simulink library "component_lib"  (R2023a)
settings: Solver=VariableStepAuto  StartTime=0.0  StopTime=10.0  RelTol=1e-3
undefined symbols (not defined in the file or in its folder): ECCV_r, par, R1234yf_ph, V_nom
libraries: base_lib x258, $bdroot x212, simulink x2, slpidlib x1
(part 5 of 7)

== system component_lib/Thermal Systems/RF0003_compressor ==
  V_bus [V] : Inport
  p2 [Pa] : Inport  Port=2
  N [rpm] : Inport  Port=3
  "RF: (h1, p1, ~)" : Inport  Port=4
  Constant : Constant  Value=W0
  Constant1 : Constant  Value=400e3
  Demux : Demux  Outputs=3
  Density Look-up : Lookup_n-D  BreakpointsForDimension1=R1234yf_ph.p  BreakpointsForDimension2=R1234yf_ph.h  Table=R1234yf_ph.D  InternalRulePriority=Speed  RndMeth=Simplest
      settings: InputPortMap=u0,u1
  Divide : Product  Inputs=*/
  Divide1 : Product  Inputs=*/
  F0021_cp.m : base_lib/F0021_R1234yf/F0021_cp.m  SystemSampleTime=-1  VariantActivationTime=update diagram  Latency=0  AutoFrameSizeCalculation=off
      settings: LibrarySourceBlock=|
      | simulink/User-Defined
      | Functions/MATLAB Function
  F0021_cv.m : base_lib/F0021_R1234yf/F0021_cv.m  SystemSampleTime=-1  VariantActivationTime=update diagram  Latency=0  AutoFrameSizeCalculation=off
      settings: LibrarySourceBlock=|
      | simulink/User-Defined
      | Functions/MATLAB Function
  F0022_compressor.m : base_lib/F0022_heatPump/F0022_compressor.m  SystemSampleTime=-1  VariantActivationTime=update diagram  Latency=0  AutoFrameSizeCalculation=off
      settings: LibrarySourceBlock=|
      | simulink/User-Defined
      | Functions/MATLAB Function
  Gain : Gain  Gain=1/60
  Gain1 : Gain  Gain=par.M
  Gain2 : Gain  Gain=1/par.M
  Gain3 : Gain  Gain=1/t_c
  Gain4 : Gain  Gain=1/t_c
  Integrator : Integrator  InitialConditionSource=external  LimitOutput=on  LowerSaturationLimit=0
  Integrator1 : Integrator  InitialConditionSource=external  LimitOutput=on  LowerSaturationLimit=0
  Mux : Mux  Inputs=3
  Negative flow barred : Saturate  UpperLimit=inf  LowerLimit=0
  Power limit : Saturate  UpperLimit=1e4  LowerLimit=0
  Saturation : Saturate  UpperLimit=par.Tc-1  LowerLimit=0
  Sum : Sum  Inputs=|+-
  Sum1 : Sum  Inputs=|+-
  Temperature Look-up : Lookup_n-D  BreakpointsForDimension1=R1234yf_ph.p  BreakpointsForDimension2=R1234yf_ph.h  Table=R1234yf_ph.T  InternalRulePriority=Speed  RndMeth=Simplest
      settings: InputPortMap=u0,u1
  Terminator : Terminator
  I [A] : Outport
  "RF: (h2, p2, W2)" : Outport  Port=2
  wires:
  Gain1/1 -> F0022_compressor.m/3, Density Look-up/2, Temperature Look-up/2
  [p_1] -> Temperature Look-up/1, Density Look-up/1, F0022_compressor.m/1
  N [rpm]/1 -> Gain/1
  F0022_compressor.m/1 -> Negative flow barred/1
  F0022_compressor.m/2 -> Power limit/1
  Density Look-up/1 -> F0022_compressor.m/2, F0021_cv.m/2, F0021_cp.m/2
  F0021_cp.m/1 -> Divide/1
  F0021_cv.m/1 -> Divide/2
  Divide/1 -> F0022_compressor.m/6
  Temperature Look-up/1 -> Saturation/1
  F0022_compressor.m/3 -> Gain2/1
  p2 [Pa]/1 -> [p_2], F0022_compressor.m/4
  Saturation/1 -> F0021_cv.m/1, F0021_cp.m/1
  Negative flow barred/1 -> Sum/1
  Gain/1 -> F0022_compressor.m/5
  Integrator/1 -> Sum/2, [W]
  [h_1] -> Gain1/1
  "RF: (h1, p1, ~)"/1 -> Demux/1
  Demux/1 -> [h_1]
  Demux/2 -> [p_1]
  Mux/1 -> "RF: (h2, p2, W2)"/1
  [h_2] -> Mux/1
  [p_2] -> Mux/2
  [W] -> Mux/3
  Demux/3 -> Terminator/1
  Sum/1 -> Gain3/1
  Gain3/1 -> Integrator/1
  Constant/1 -> Integrator/2
  Gain2/1 -> Sum1/1
  Sum1/1 -> Gain4/1
  Integrator1/1 -> Sum1/2, [h_2]
  Gain4/1 -> Integrator1/1
  Constant1/1 -> Integrator1/2
  V_bus [V]/1 -> Divide1/2
  Power limit/1 -> Divide1/1
  Divide1/1 -> I [A]/1

== system component_lib/Thermal Systems/RF0004_smoothTube ==
  "RF: (h1, p1, W1)" : Inport
  Abs : Abs  SaturateOnIntegerOverflow=off
  Demux : Demux  Outputs=3
  F0021_dliqsat.m : base_lib/F0021_R1234yf/F0021_dliqsat.m  SystemSampleTime=-1  VariantActivationTime=update diagram  Latency=0  AutoFrameSizeCalculation=off
      settings: LibrarySourceBlock=|
      | simulink/User-Defined
      | Functions/MATLAB Function
  F0021_dvapsat.m : base_lib/F0021_R1234yf/F0021_dvapsat.m  SystemSampleTime=-1  VariantActivationTime=update diagram  Latency=0  AutoFrameSizeCalculation=off
      settings: LibrarySourceBlock=|
      | simulink/User-Defined
      | Functions/MATLAB Function
  F0022_smoothTubePressureDrop.m : base_lib/F0022_heatPump/F0022_smoothTubePressureDrop.m  SystemSampleTime=-1  VariantActivationTime=update diagram  Latency=0  AutoFrameSizeCalculation=off
      settings: LibrarySourceBlock=|
      | simulink/User-Defined
      | Functions/MATLAB Function
  Gain{2,4..5,7} (4 alike) : Gain  Gain=par.M
  Mux : Mux  Inputs=3
  R1234yf_mu.m : base_lib/F0021_R1234yf/R1234yf_mu.m  SystemSampleTime=-1  VariantActivationTime=update diagram  Latency=0  AutoFrameSizeCalculation=off
      settings: LibrarySourceBlock=|
      | simulink/User-Defined
      | Functions/MATLAB Function
  R1234yf_mu.m1 : base_lib/F0021_R1234yf/R1234yf_mu.m  SystemSampleTime=-1  VariantActivationTime=update diagram  Latency=0  AutoFrameSizeCalculation=off
      settings: LibrarySourceBlock=|
      | simulink/User-Defined
      | Functions/MATLAB Function
  R1234yf_sigma.m : base_lib/F0021_R1234yf/R1234yf_sigma.m  SystemSampleTime=-1  VariantActivationTime=update diagram  Latency=0  AutoFrameSizeCalculation=off
      settings: LibrarySourceBlock=|
      | simulink/User-Defined
      | Functions/MATLAB Function
  Saturation : Saturate  UpperLimit=par.Tc-1  LowerLimit=0
  Saturation1 : Saturate  UpperLimit=1  LowerLimit=0
  Sum : Sum  Inputs=|+-
  Temperature Look-up : Lookup_n-D  BreakpointsForDimension1=R1234yf_ph.p  BreakpointsForDimension2=R1234yf_ph.h  Table=R1234yf_ph.T  InternalRulePriority=Speed  RndMeth=Simplest
      settings: InputPortMap=u0,u1
  Vapor Fraction Look-up : Lookup_n-D  BreakpointsForDimension1=R1234yf_ph.p  BreakpointsForDimension2=R1234yf_ph.h  Table=R1234yf_ph.x  InternalRulePriority=Speed  RndMeth=Simplest
      settings: InputPortMap=u0,u1
  "RF: (h2, p2, W2)" : Outport
  wires:
  Gain2/1 -> Temperature Look-up/2
  [W1] -> Abs/1
  Gain4/1 -> Vapor Fraction Look-up/2
  Vapor Fraction Look-up/1 -> Saturation1/1
  F0021_dvapsat.m/1 -> R1234yf_mu.m1/2, Gain5/1
  Temperature Look-up/1 -> Saturation/1
  Gain5/1 -> F0022_smoothTubePressureDrop.m/4
  F0021_dliqsat.m/1 -> R1234yf_mu.m/2, Gain7/1
  Gain7/1 -> F0022_smoothTubePressureDrop.m/3
  R1234yf_mu.m/1 -> F0022_smoothTubePressureDrop.m/5
  R1234yf_mu.m1/1 -> F0022_smoothTubePressureDrop.m/6
  R1234yf_sigma.m/1 -> F0022_smoothTubePressureDrop.m/7
  [h1] -> Gain4/1, Gain2/1
  Abs/1 -> F0022_smoothTubePressureDrop.m/1
  Demux/2 -> [p1]
  "RF: (h1, p1, W1)"/1 -> Demux/1
  [p1] -> Sum/1
  Sum/1 -> [p2]
  [p1] -> Temperature Look-up/1, Vapor Fraction Look-up/1
  F0022_smoothTubePressureDrop.m/1 -> Sum/2
  Saturation/1 -> R1234yf_sigma.m/1, R1234yf_mu.m1/1, R1234yf_mu.m/1, F0021_dvapsat.m/1, F0021_dliqsat.m/1
  Saturation1/1 -> F0022_smoothTubePressureDrop.m/2
  Mux/1 -> "RF: (h2, p2, W2)"/1
  Demux/1 -> [h1]
  Demux/3 -> [W1]
  [h1] -> Mux/1
  [W1] -> Mux/3
  [p2] -> Mux/2

== system component_lib/Thermal Systems/RF0005_expansionValve ==
  exv [-] : Inport
  "RF: (h1, p1, W)" : Inport  Port=2
  Demux : Demux  Outputs=3
  Density Look-up : Lookup_n-D  BreakpointsForDimension1=R1234yf_ph.p  BreakpointsForDimension2=R1234yf_ph.h  Table=R1234yf_ph.D  InternalRulePriority=Speed  RndMeth=Simplest
      settings: InputPortMap=u0,u1
  F0021_Tsat.m : base_lib/F0021_R1234yf/F0021_Tsat.m  SystemSampleTime=-1  VariantActivationTime=update diagram  Latency=0  AutoFrameSizeCalculation=off
      settings: LibrarySourceBlock=|
      | simulink/User-Defined
      | Functions/MATLAB Function
  F0022_expansionValve.m : base_lib/F0022_heatPump/F0022_expansionValve.m  SystemSampleTime=-1  VariantActivationTime=update diagram  Latency=0  AutoFrameSizeCalculation=off
      settings: LibrarySourceBlock=|
      | simulink/User-Defined
      | Functions/MATLAB Function
  Gain1 : Gain  Gain=par.M
  Gain2 : Gain  Gain=par.M
  Gain6 : Gain  Gain=par.M
  Mux : Mux  Inputs=3
  Saturation : Saturate  UpperLimit=1  LowerLimit=0
  Saturation1 : Saturate  UpperLimit=par.Tc-1  LowerLimit=0
  Saturation2 : Saturate  UpperLimit=par.pc  LowerLimit=0
  Saturation3 : Saturate  UpperLimit=inf  LowerLimit=p_min
  Sum : Sum  Inputs=|+-
  Temperature Look-up : Lookup_n-D  BreakpointsForDimension1=R1234yf_ph.p  BreakpointsForDimension2=R1234yf_ph.h  Table=R1234yf_ph.T  InternalRulePriority=Speed  RndMeth=Simplest
      settings: InputPortMap=u0,u1
  Transfer Fcn : TransferFcn  Denominator=[1 1]
  dp [Pa] : Outport
  "RF: (h2, p2, W2)" : Outport  Port=2
  wires:
  Gain2/1 -> Temperature Look-up/2
  Gain1/1 -> Density Look-up/2
  Density Look-up/1 -> Gain6/1
  [h_1] -> Gain1/1, Gain2/1
  exv [-]/1 -> Saturation/1
  F0021_Tsat.m/1 -> F0022_expansionValve.m/5
  Gain6/1 -> F0022_expansionValve.m/4
  Saturation/1 -> F0022_expansionValve.m/6
  Temperature Look-up/1 -> Saturation1/1
  Saturation1/1 -> F0022_expansionValve.m/3
  Saturation2/1 -> F0021_Tsat.m/1
  [p_1] -> Saturation2/1, Density Look-up/1, Temperature Look-up/1, F0022_expansionValve.m/2
  F0022_expansionValve.m/1 -> dp [Pa]/1, Transfer Fcn/1
  "RF: (h1, p1, W)"/1 -> Demux/1
  Demux/2 -> [p_1]
  Demux/3 -> [W]
  Demux/1 -> [h2], [h_1]
  [W] -> F0022_expansionValve.m/1
  Mux/1 -> "RF: (h2, p2, W2)"/1
  [W] -> Mux/3
  [h2] -> Mux/1
  Transfer Fcn/1 -> Sum/2
  [p_1] -> Sum/1
  Sum/1 -> Saturation3/1
  Saturation3/1 -> Mux/2

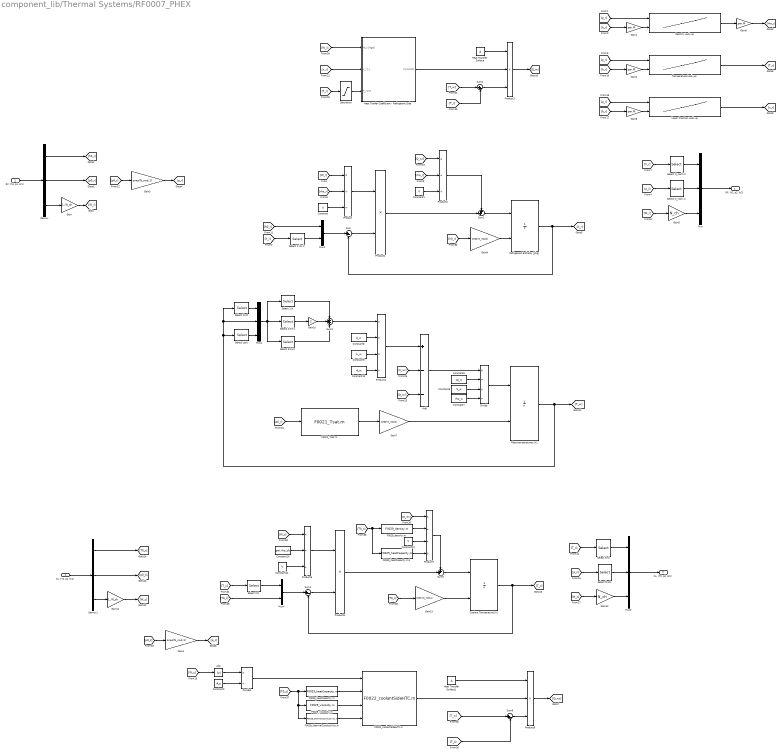
== system component_lib/Thermal Systems/RF0007_PHEX ==
  "RF: (h1, p1, W1)" : Inport
  "CL: (T1, p1, W1)" : Inport  Port=2
  Abs : Abs  SaturateOnIntegerOverflow=off
  Add : Sum  Inputs=+--
  Constant{,1,11..12} (4 alike) : Constant  Value=V
  Constant10 : Constant  Value=d_w
  Constant14 : Constant  Value=par.rho_clt
  Constant2 : Constant  Value=A_c
  Constant5 : Constant  Value=cp_w
  Constant6 : Constant  Value=V_w
  Constant7 : Constant  Value=rho_w
  Constant8 : Constant  Value=A_w
  Constant9 : Constant  Value=k_w
  Coolant Temperature [K] : Integrator  InitialConditionSource=external  LimitOutput=on  LowerSaturationLimit=0
  Demux : Demux  Outputs=3
  Demux1 : Demux  Outputs=3
  Density Look-up : Lookup_n-D  BreakpointsForDimension1=R1234yf_ph.p  BreakpointsForDimension2=R1234yf_ph.h  Table=R1234yf_ph.D  InternalRulePriority=Speed  RndMeth=Simplest
      settings: InputPortMap=u0,u1
  Divide : Product  Inputs=*///
  Divide1 : Product  Inputs=*/
  F0021_Tsat.m : base_lib/F0021_R1234yf/F0021_Tsat.m  SystemSampleTime=-1  VariantActivationTime=update diagram  Latency=0  AutoFrameSizeCalculation=off
      settings: LibrarySourceBlock=|
      | simulink/User-Defined
      | Functions/MATLAB Function
  F0022_coolantSideHTC.m : base_lib/F0022_heatPump/F0022_coolantSideHTC.m  SystemSampleTime=-1  VariantActivationTime=update diagram  Latency=0  AutoFrameSizeCalculation=off
      settings: LibrarySourceBlock=|
      | simulink/User-Defined
      | Functions/MATLAB Function
  F0029_density.m : base_lib/F0029_coolantWrapper/F0029_density.m  SystemSampleTime=-1  VariantActivationTime=update diagram  Latency=0  AutoFrameSizeCalculation=off
      settings: LibrarySourceBlock=|
      | simulink/User-Defined
      | Functions/MATLAB Function
  F0029_heatCapacity.m : base_lib/F0029_coolantWrapper/F0029_heatCapacity.m  SystemSampleTime=-1  VariantActivationTime=update diagram  Latency=0  AutoFrameSizeCalculation=off
      settings: LibrarySourceBlock=|
      | simulink/User-Defined
      | Functions/MATLAB Function
  F0029_heatCapacity.m1 : base_lib/F0029_coolantWrapper/F0029_heatCapacity.m  SystemSampleTime=-1  VariantActivationTime=update diagram  Latency=0  AutoFrameSizeCalculation=off
      settings: LibrarySourceBlock=|
      | simulink/User-Defined
      | Functions/MATLAB Function
  F0029_thermalConductivity.m : base_lib/F0029_coolantWrapper/F0029_thermalConductivity.m  SystemSampleTime=-1  VariantActivationTime=update diagram  Latency=0  AutoFrameSizeCalculation=off
      settings: LibrarySourceBlock=|
      | simulink/User-Defined
      | Functions/MATLAB Function
  F0029_viscosity.m : base_lib/F0029_coolantWrapper/F0029_viscosity.m  SystemSampleTime=-1  VariantActivationTime=update diagram  Latency=0  AutoFrameSizeCalculation=off
      settings: LibrarySourceBlock=|
      | simulink/User-Defined
      | Functions/MATLAB Function
  Gain : Gain  Gain=1./N_ch
  Gain{1..2,6,8} (4 alike) : Gain  Gain=par.M
  Gain10 : Gain  Gain=2
  Gain11 : Gain  Gain=1./N_ch
  Gain12 : Gain  Gain=N_ch
  Gain{3..4,7,9,13} (5 alike) : Gain  Gain=ones(N_nod,1)
  Gain5 : Gain  Gain=N_ch
  Heat Tranfer Coefficient - Refrigerant Side : Subsystem
  Heat Transfer Surface : Constant  Value=A
  Heat Transfer Surface1 : Constant  Value=A
  Mux : Mux  Inputs=3
  Mux1 : Mux  Inputs=2
  Mux2 : Mux  Inputs=3
  Mux3 : Mux  Inputs=3
  Mux4 : Mux  Inputs=2
  Plate temperatures [K] : Integrator  InitialConditionSource=external  LimitOutput=on  LowerSaturationLimit=0
  Product : Product  Inputs=*//
  Product1 : Product
  Product2 : Product  Inputs=*//
  Product3 : Product  Inputs=3
  Product4 : Product  Inputs=***/
  Product5 : Product  Inputs=*//
  Product6 : Product
  Product7 : Product  Inputs=*///
  Product8 : Product  Inputs=3
  Refrigerant Enthalpy [J/kg] : Integrator  InitialConditionSource=external  LimitOutput=on  LowerSaturationLimit=0
  Saturation : Saturate  UpperLimit=par.Tc-2  LowerLimit=0
  Select 1:(N-1) : Selector  InputPortWidth=N_nod  IndexOptions=Index vector (dialog)  Indices=[1:(N_nod-1)]  OutputSizes=1
  Select 1:N : Selector  InputPortWidth=N_nod+2  IndexOptions=Index vector (dialog)  Indices=[1:N_nod]  OutputSizes=1
  Select 2:N : Selector  InputPortWidth=N_nod  IndexOptions=Index vector (dialog)  Indices=[2:N_nod]  OutputSizes=1
  "Select 2:N+1 " : Selector  InputPortWidth=N_nod+2  IndexOptions=Index vector (dialog)  Indices=[2:(N_nod+1)]  OutputSizes=1
  Select 3:N+2 : Selector  InputPortWidth=N_nod+2  IndexOptions=Index vector (dialog)  Indices=[3:(N_nod+2)]  OutputSizes=1
  Select First : Selector  InputPortWidth=N_nod  IndexOptions=Index vector (dialog)  Indices=1  OutputSizes=1
  Select Last : Selector  InputPortWidth=N_nod  IndexOptions=Index vector (dialog)  Indices=N_nod  OutputSizes=1
  Select N_nod (1) : Selector  InputPortWidth=N_nod  IndexOptions=Index vector (dialog)  Indices=N_nod  OutputSizes=1
  Select N_nod (2) : Selector  InputPortWidth=N_nod  IndexOptions=Index vector (dialog)  Indices=N_nod  OutputSizes=1
  Select first : Selector  InputPortWidth=N_nod  IndexOptions=Index vector (dialog)  Indices=1  OutputSizes=1
  Select first1 : Selector  InputPortWidth=N_nod  IndexOptions=Index vector (dialog)  Indices=1  OutputSizes=1
  Sum{,2,4,6} (4 alike) : Sum  Inputs=|+-
  Sum1 : Sum  Inputs=++|
  Sum3 : Sum  Inputs=+-+
  Sum5 : Sum  Inputs=++|
  Temperature Look-up : Lookup_n-D  BreakpointsForDimension1=R1234yf_ph.p  BreakpointsForDimension2=R1234yf_ph.h  Table=R1234yf_ph.T  InternalRulePriority=Speed  RndMeth=Simplest
      settings: InputPortMap=u0,u1
  Vapor Fraction Look-up : Lookup_n-D  BreakpointsForDimension1=R1234yf_ph.p  BreakpointsForDimension2=R1234yf_ph.h  Table=R1234yf_ph.x  InternalRulePriority=Speed  RndMeth=Simplest
      settings: InputPortMap=u0,u1
  "RF: (h2, p2, W2)" : Outport
  "CL: (T2, p2, W2)" : Outport  Port=2
  wires:
  [h_r] -> Gain1/1
  Demux/2 -> [p0_r]
  "RF: (h1, p1, W1)"/1 -> Demux/1
  Mux/1 -> "RF: (h2, p2, W2)"/1
  [W_r] -> Gain5/1
  [p_r] -> Select N_nod (1)/1
  Density Look-up/1 -> Gain6/1
  Gain1/1 -> Density Look-up/2
  Gain6/1 -> [rho_r]
  Constant/1 -> Product/3
  [rho_r] -> Product/2
  [W_r] -> Product/1
  Product/1 -> Product1/1
  Sum/1 -> Product1/2
  Product1/1 -> Sum1/2
  Sum1/1 -> Refrigerant Enthalpy [J/kg]/1
  Constant1/1 -> Product2/3
  [rho_r] -> Product2/2
  Product2/1 -> Sum1/1
  Gain9/1 -> Refrigerant Enthalpy [J/kg]/2
  Refrigerant Enthalpy [J/kg]/1 -> [h_r], Sum/2
  [h_r] -> Select 1:(N-1)/1
  Select 1:(N-1)/1 -> Mux1/2
  [h0_r] -> Mux1/1
  [p_r] -> Density Look-up/1
  [p0_r] -> Gain3/1
  Gain3/1 -> [p_r]
  [h_r] -> Select N_nod (2)/1
  Select N_nod (1)/1 -> Mux/2
  Mux1/1 -> Sum/1
  [h_r] -> Gain2/1
  Gain2/1 -> Temperature Look-up/2
  [p_r] -> Temperature Look-up/1
  [Q_wr] -> Product2/1
  [h_r] -> Gain8/1
  [p_r] -> Vapor Fraction Look-up/1
  Gain8/1 -> Vapor Fraction Look-up/2
  Vapor Fraction Look-up/1 -> [x_r]
  Gain/1 -> [W_r]
  Gain7/1 -> Plate temperatures [K]/2
  Divide/1 -> Plate temperatures [K]/1
  Add/1 -> Divide/1
  Constant5/1 -> Divide/2
  Constant6/1 -> Divide/3
  Constant7/1 -> Divide/4
  [Q_wr] -> Add/3
  Plate temperatures [K]/1 -> [T_w], Select First/1, Mux2/2, Select Last/1
  Select First/1 -> Mux2/1
  Mux2/1 -> Select 3:N+2/1, "Select 2:N+1 "/1, Select 1:N/1
  Select Last/1 -> Mux2/3
  "Select 2:N+1 "/1 -> Gain10/1
  Gain10/1 -> Sum3/2
  Select 1:N/1 -> Sum3/1
  Select 3:N+2/1 -> Sum3/3
  Sum3/1 -> Product4/1
  Constant8/1 -> Product4/2
  Constant9/1 -> Product4/3
  Constant10/1 -> Product4/4
  Product4/1 -> Add/1
  [Q_wc] -> Add/2
  Gain11/1 -> [W_c]
  Demux1/2 -> [p0_c]
  "CL: (T1, p1, W1)"/1 -> Demux1/1
  [T_c] -> Select first/1
  Select first1/1 -> Mux3/2
  [W_c] -> Gain12/1
  Mux3/1 -> "CL: (T2, p2, W2)"/1
  [p_c] -> Select first1/1
  [Q_wc] -> Product7/1
  Mux4/1 -> Sum4/1
  Coolant Temperature [K]/1 -> [T_c], Sum4/2
  Product7/1 -> Sum5/1
  Gain13/1 -> Coolant Temperature [K]/2
  [T_c] -> Select 2:N/1
  Sum5/1 -> Coolant Temperature [K]/1
  Sum4/1 -> Product6/2
  Product5/1 -> Product6/1
  [W_c] -> Product5/1
  Product6/1 -> Sum5/2
  [W_r] -> Heat Tranfer Coefficient - Refrigerant Side/1(W_r [kg/s])
  [x_r] -> Heat Tranfer Coefficient - Refrigerant Side/2(x_r [-])
  [T_r] -> Saturation/1
  Heat Transfer Surface/1 -> Product3/1
  [T_w] -> Sum2/1
  Sum2/1 -> Product3/3
  [T_r] -> Sum2/2
  Product3/1 -> [Q_wr]
  Heat Tranfer Coefficient - Refrigerant Side/1(h [W/mK]) -> Product3/2
  F0029_heatCapacity.m1/1 -> Product7/4
  Constant14/1 -> Product5/2
  Divide1/1 -> F0022_coolantSideHTC.m/1
  Product8/1 -> [Q_wc]
  F0022_coolantSideHTC.m/1 -> Product8/2
  Sum6/1 -> Product8/3
  [T_c] -> Sum6/2
  Temperature Look-up/1 -> [T_r]
  Gain4/1 -> [p_c]
  [p0_c] -> Gain4/1
  Saturation/1 -> Heat Tranfer Coefficient - Refrigerant Side/3(T_r [K])
  [T_w] -> Sum6/1
  Heat Transfer Surface1/1 -> Product8/1
  Constant11/1 -> Product5/3
  Constant12/1 -> Product7/3
  [T0_c] -> Mux4/2
  Select 2:N/1 -> Mux4/1
  Demux/3 -> Gain/1
  Demux/1 -> [h0_r]
  Gain5/1 -> Mux/3
  Select N_nod (2)/1 -> Mux/1
  Gain12/1 -> Mux3/3
  Select first/1 -> Mux3/1
  Demux1/3 -> Gain11/1
  Demux1/1 -> [T0_c]
  F0021_Tsat.m/1 -> Gain7/1
  [p0_r] -> F0021_Tsat.m/1
  [h0_r] -> Gain9/1
  [T0_c] -> Gain13/1
  Abs/1 -> Divide1/1
  Constant2/1 -> Divide1/2
  [W_c] -> Abs/1
  F0029_heatCapacity.m/1 -> F0022_coolantSideHTC.m/2
  F0029_viscosity.m/1 -> F0022_coolantSideHTC.m/3
  F0029_thermalConductivity.m/1 -> F0022_coolantSideHTC.m/4
  [T0_c] -> F0029_thermalConductivity.m/1, F0029_viscosity.m/1, F0029_heatCapacity.m/1
  F0029_density.m/1 -> Product7/2
  [T0_c] -> F0029_heatCapacity.m1/1, F0029_density.m/1

== system component_lib/Thermal Systems/RF0008_receiver_old ==
  "RF: (h1, ~, W)" : Inport
  Constant1 : Constant  Value=V
  Constant4 : Constant  Value=h0
  Demux : Demux  Outputs=3
  Density Look-up : Lookup_n-D  BreakpointsForDimension1=R1234yf_ph.p  BreakpointsForDimension2=R1234yf_ph.h  Table=R1234yf_ph.D  InternalRulePriority=Speed  RndMeth=Simplest
      settings: InputPortMap=u0,u1
  Divide : Product  Inputs=*/
  F0021_dliqsat.m1 : base_lib/F0021_R1234yf/F0021_dliqsat.m  SystemSampleTime=-1  VariantActivationTime=update diagram  Latency=0  AutoFrameSizeCalculation=off
      settings: LibrarySourceBlock=|
      | simulink/User-Defined
      | Functions/MATLAB Function
  F0021_h.m1 : base_lib/F0021_R1234yf/F0021_h.m  SystemSampleTime=-1  VariantActivationTime=update diagram  Latency=0  AutoFrameSizeCalculation=off
      settings: LibrarySourceBlock=|
      | simulink/User-Defined
      | Functions/MATLAB Function
  Gain1 : Gain  Gain=1/par.M
  Gain{3..5,16} (4 alike) : Gain  Gain=par.M
  Gain2 : Gain  Gain=1/par.M
  Min : MinMax  Inputs=2
  Mux : Mux  Inputs=3
  Product1 : Product
  Product2 : Product
  Product3 : Product
  Specific Enthalpy [J/kg] : Integrator  InitialConditionSource=external  LimitOutput=on  LowerSaturationLimit=0
  Sum3 : Sum  Inputs=+|-
  Temperature Look-up : Lookup_n-D  BreakpointsForDimension1=R1234yf_ph.p  BreakpointsForDimension2=R1234yf_ph.h  Table=R1234yf_ph.T  InternalRulePriority=Speed  RndMeth=Simplest
      settings: InputPortMap=u0,u1
  "RF: (h2, p2, W)" : Outport
  wires:
  F0021_h.m1/1 -> Gain1/1
  Gain2/1 -> F0021_h.m1/2
  [rho_f] -> Gain2/1
  [T] -> F0021_dliqsat.m1/1, F0021_h.m1/1
  F0021_dliqsat.m1/1 -> Gain16/1
  Gain16/1 -> [rho_f]
  [h_1] -> Product2/2
  [W] -> Product2/1
  Product2/1 -> Sum3/1
  [h_f] -> Product3/2
  Product3/1 -> Sum3/2
  [W] -> Product3/1
  Specific Enthalpy [J/kg]/1 -> [h]
  [h] -> Gain4/1
  Temperature Look-up/1 -> [T]
  Gain4/1 -> Temperature Look-up/2
  [p] -> Temperature Look-up/1
  Constant1/1 -> Product1/2
  [rho] -> Product1/1
  Density Look-up/1 -> Gain5/1
  Gain3/1 -> Density Look-up/2
  [p] -> Density Look-up/1
  [h] -> Gain3/1
  Gain5/1 -> [rho]
  Divide/1 -> Specific Enthalpy [J/kg]/1
  Sum3/1 -> Divide/1
  Product1/1 -> Divide/2
  Constant4/1 -> Specific Enthalpy [J/kg]/2
  Mux/1 -> "RF: (h2, p2, W)"/1
  [p] -> Mux/2
  [W] -> Mux/3
  "RF: (h1, ~, W)"/1 -> Demux/1
  Demux/1 -> [h_1]
  Demux/3 -> [W]
  [h_f] -> Mux/1
  Demux/2 -> [p]
  Min/1 -> [h_f]
  Gain1/1 -> Min/1
  [h] -> Min/2

== system component_lib/Thermal Systems/RF0010_calculateSuperHeat ==
  "RF: (h, p, W)" : Inport
  Demux : Demux  Outputs=3
  F0021_Tsat.m : base_lib/F0021_R1234yf/F0021_Tsat.m  SystemSampleTime=-1  VariantActivationTime=update diagram  Latency=0  AutoFrameSizeCalculation=off
      settings: LibrarySourceBlock=|
      | simulink/User-Defined
      | Functions/MATLAB Function
  Gain2 : Gain  Gain=par.M
  Saturation : Saturate  UpperLimit=inf  LowerLimit=0
  Sum : Sum  Inputs=|+-
  Temperature Look-up : Lookup_n-D  BreakpointsForDimension1=R1234yf_ph.p  BreakpointsForDimension2=R1234yf_ph.h  Table=R1234yf_ph.T  InternalRulePriority=Speed  RndMeth=Simplest
      settings: InputPortMap=u0,u1
  T_sup [K] : Outport
  wires:
  Demux/2 -> [p]
  Gain2/1 -> Temperature Look-up/2
  [p] -> F0021_Tsat.m/1, Temperature Look-up/1
  [h] -> Gain2/1
  Temperature Look-up/1 -> Sum/1
  F0021_Tsat.m/1 -> Sum/2
  Sum/1 -> Saturation/1
  Saturation/1 -> T_sup [K]/1
  "RF: (h, p, W)"/1 -> Demux/1
  Demux/1 -> [h]
  Demux/3 -> [W]

== system component_lib/Thermal Systems/RF0011_calculateSubCool ==
  "RF: (h, p, W)" : Inport
  Demux : Demux  Outputs=3
  F0021_Tsat.m : base_lib/F0021_R1234yf/F0021_Tsat.m  SystemSampleTime=-1  VariantActivationTime=update diagram  Latency=0  AutoFrameSizeCalculation=off
      settings: LibrarySourceBlock=|
      | simulink/User-Defined
      | Functions/MATLAB Function
  Gain2 : Gain  Gain=par.M
  Saturation : Saturate  UpperLimit=inf  LowerLimit=0
  Sum : Sum  Inputs=|+-
  Temperature Look-up : Lookup_n-D  BreakpointsForDimension1=R1234yf_ph.p  BreakpointsForDimension2=R1234yf_ph.h  Table=R1234yf_ph.T  InternalRulePriority=Speed  RndMeth=Simplest
      settings: InputPortMap=u0,u1
  T_sub [K] : Outport
  wires:
  "RF: (h, p, W)"/1 -> Demux/1
  Demux/2 -> [p]
  Gain2/1 -> Temperature Look-up/2
  [p] -> F0021_Tsat.m/1, Temperature Look-up/1
  [h] -> Gain2/1
  Sum/1 -> Saturation/1
  F0021_Tsat.m/1 -> Sum/1
  Temperature Look-up/1 -> Sum/2
  Saturation/1 -> T_sub [K]/1
  Demux/1 -> [h]
  Demux/3 -> [W]

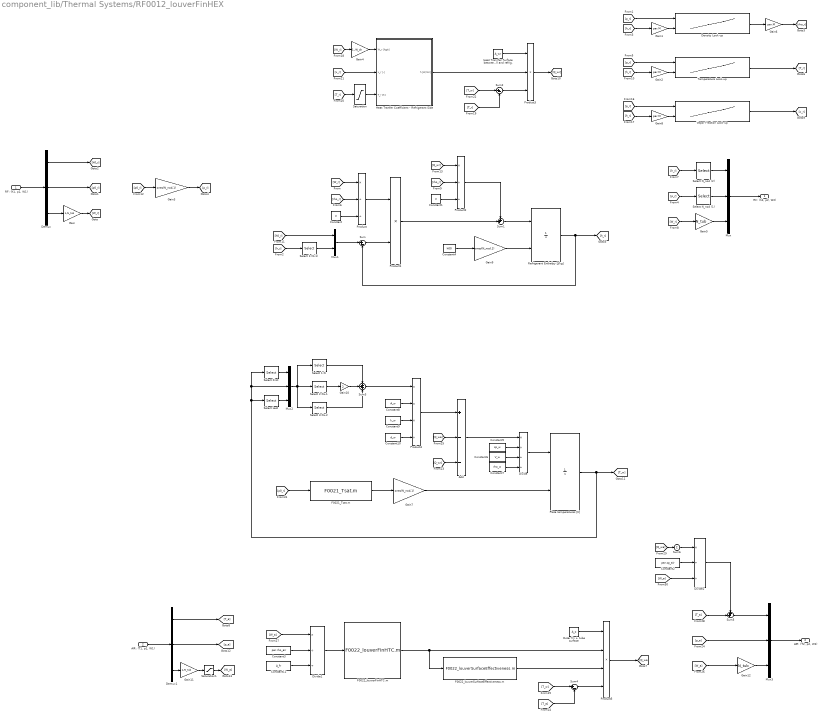
== system component_lib/Thermal Systems/RF0012_louverFinHEX ==
  "RF: (h1, p1, W1)" : Inport
  "AIR: (T1, p1, W1)" : Inport  Port=2
  Add : Sum  Inputs=+--
  Constant : Constant  Value=V
  Constant1 : Constant  Value=V
  Constant10 : Constant  Value=d_w
  Constant11 : Constant  Value=A_fr
  Constant2 : Constant  Value=par.cp_air
  Constant3 : Constant  Value=par.rho_air
  Constant4 : Constant  Value=h00
  Constant5 : Constant  Value=cp_w
  Constant6 : Constant  Value=V_w
  Constant7 : Constant  Value=rho_w
  Constant8 : Constant  Value=A_w
  Constant9 : Constant  Value=k_w
  Demux : Demux  Outputs=3
  Demux1 : Demux  Outputs=3
  Density Look-up : Lookup_n-D  BreakpointsForDimension1=R1234yf_ph.p  BreakpointsForDimension2=R1234yf_ph.h  Table=R1234yf_ph.D  InternalRulePriority=Speed  RndMeth=Simplest
      settings: InputPortMap=u0,u1
  Divide : Product  Inputs=*///
  Divide1 : Product  Inputs=*//
  Divide2 : Product  Inputs=*//
  F0021_Tsat.m : base_lib/F0021_R1234yf/F0021_Tsat.m  SystemSampleTime=-1  VariantActivationTime=update diagram  Latency=0  AutoFrameSizeCalculation=off
      settings: LibrarySourceBlock=|
      | simulink/User-Defined
      | Functions/MATLAB Function
  F0022_louverFinHTC.m : base_lib/F0022_heatPump/F0022_louverFinHTC.m  SystemSampleTime=-1  VariantActivationTime=update diagram  Latency=0  AutoFrameSizeCalculation=off
      settings: LibrarySourceBlock=|
      | simulink/User-Defined
      | Functions/MATLAB Function
  F0022_louverSurfaceEffectiveness.m : base_lib/F0022_heatPump/F0022_louverSurfaceEffectiveness.m  SystemSampleTime=-1  VariantActivationTime=update diagram  Latency=0  AutoFrameSizeCalculation=off
      settings: LibrarySourceBlock=|
      | simulink/User-Defined
      | Functions/MATLAB Function
  Gain : Gain  Gain=1./N_tub
  Gain{1..2,6,8} (4 alike) : Gain  Gain=par.M
  Gain10 : Gain  Gain=2
  Gain11 : Gain  Gain=1./N_tub
  Gain12 : Gain  Gain=N_tub
  Gain3 : Gain  Gain=ones(N_nod,1)
  Gain4 : Gain  Gain=1./N_ch
  Gain5 : Gain  Gain=N_tub
  Gain7 : Gain  Gain=ones(N_nod,1)
  Gain9 : Gain  Gain=ones(N_nod,1)
  Heat Tranfer Coefficient - Refrigerant Side : Subsystem
  Heat Transfer Surface between wall and refrig. : Constant  Value=A_wr
  Mux : Mux  Inputs=3
  Mux1 : Mux  Inputs=2
  Mux2 : Mux  Inputs=3
  Mux3 : Mux  Inputs=3
  Outer fin + tube surface : Constant  Value=A_o
  Plate temperatures [K] : Integrator  InitialConditionSource=external  LimitOutput=on  LowerSaturationLimit=0
  Product : Product  Inputs=*//
  Product1 : Product
  Product2 : Product  Inputs=*//
  Product3 : Product  Inputs=3
  Product4 : Product  Inputs=***/
  Product5 : Product  Inputs=4
  Refrigerant Enthalpy [J/kg] : Integrator  InitialConditionSource=external  LimitOutput=on  LowerSaturationLimit=0
  Saturation : Saturate  UpperLimit=par.Tc-2  LowerLimit=0
  Saturation1 : Saturate  UpperLimit=inf  LowerLimit=1e-5
  Select 1:(N-1) : Selector  InputPortWidth=N_nod  IndexOptions=Index vector (dialog)  Indices=[1:(N_nod-1)]  OutputSizes=1
  Select 1:N : Selector  InputPortWidth=N_nod+2  IndexOptions=Index vector (dialog)  Indices=[1:N_nod]  OutputSizes=1
  "Select 2:N+1 " : Selector  InputPortWidth=N_nod+2  IndexOptions=Index vector (dialog)  Indices=[2:(N_nod+1)]  OutputSizes=1
  Select 3:N+2 : Selector  InputPortWidth=N_nod+2  IndexOptions=Index vector (dialog)  Indices=[3:(N_nod+2)]  OutputSizes=1
  Select First : Selector  InputPortWidth=N_nod  IndexOptions=Index vector (dialog)  Indices=1  OutputSizes=1
  Select Last : Selector  InputPortWidth=N_nod  IndexOptions=Index vector (dialog)  Indices=N_nod  OutputSizes=1
  Select N_nod (1) : Selector  InputPortWidth=N_nod  IndexOptions=Index vector (dialog)  Indices=N_nod  OutputSizes=1
  Select N_nod (2) : Selector  InputPortWidth=N_nod  IndexOptions=Index vector (dialog)  Indices=N_nod  OutputSizes=1
  Sum : Sum  Inputs=|+-
  Sum1 : Sum  Inputs=++|
  Sum2 : Sum  Inputs=|+-
  Sum3 : Sum  Inputs=+-+
  Sum4 : Sum  Inputs=|+-
  Sum5 : Sum  Inputs=++|
  Sum6 : Sum  Inputs=+
  Temperature Look-up : Lookup_n-D  BreakpointsForDimension1=R1234yf_ph.p  BreakpointsForDimension2=R1234yf_ph.h  Table=R1234yf_ph.T  InternalRulePriority=Speed  RndMeth=Simplest
      settings: InputPortMap=u0,u1
  Vapor Fraction Look-up : Lookup_n-D  BreakpointsForDimension1=R1234yf_ph.p  BreakpointsForDimension2=R1234yf_ph.h  Table=R1234yf_ph.x  InternalRulePriority=Speed  RndMeth=Simplest
      settings: InputPortMap=u0,u1
  "RF: (h2, p2, W2)" : Outport
  "AIR: (T2, p2, W2)" : Outport  Port=2
  wires:
  Select N_nod (2)/1 -> Mux/1
  Gain5/1 -> Mux/3
  Demux/1 -> [h0_r]
  Demux/3 -> Gain/1
  Saturation/1 -> Heat Tranfer Coefficient - Refrigerant Side/3(T_r [K])
  Temperature Look-up/1 -> [T_r]
  Heat Tranfer Coefficient - Refrigerant Side/1(h [W/mK]) -> Product3/2
  Product3/1 -> [Q_wr]
  [T_r] -> Sum2/2
  Sum2/1 -> Product3/3
  [T_w] -> Sum2/1
  Heat Transfer Surface between wall and refrig./1 -> Product3/1
  [T_r] -> Saturation/1
  [x_r] -> Heat Tranfer Coefficient - Refrigerant Side/2(x_r [-])
  Mux3/1 -> "AIR: (T2, p2, W2)"/1
  "AIR: (T1, p1, W1)"/1 -> Demux1/1
  [Q_wa] -> Add/2
  Product4/1 -> Add/1
  Constant10/1 -> Product4/4
  Constant8/1 -> Product4/2
  Sum3/1 -> Product4/1
  Select 3:N+2/1 -> Sum3/3
  Select 1:N/1 -> Sum3/1
  Gain10/1 -> Sum3/2
  "Select 2:N+1 "/1 -> Gain10/1
  Select Last/1 -> Mux2/3
  Mux2/1 -> Select 1:N/1, "Select 2:N+1 "/1, Select 3:N+2/1
  Select First/1 -> Mux2/1
  Plate temperatures [K]/1 -> Mux2/2, Select First/1, Select Last/1, [T_w]
  [Q_wr] -> Add/3
  Constant7/1 -> Divide/4
  Constant6/1 -> Divide/3
  Constant5/1 -> Divide/2
  Add/1 -> Divide/1
  Divide/1 -> Plate temperatures [K]/1
  Gain7/1 -> Plate temperatures [K]/2
  Gain/1 -> [W_r]
  Vapor Fraction Look-up/1 -> [x_r]
  Gain8/1 -> Vapor Fraction Look-up/2
  [p_r] -> Vapor Fraction Look-up/1
  [h_r] -> Gain8/1
  [Q_wr] -> Product2/1
  [p_r] -> Temperature Look-up/1
  Gain2/1 -> Temperature Look-up/2
  [h_r] -> Gain2/1
  Mux1/1 -> Sum/1
  Select N_nod (1)/1 -> Mux/2
  [h_r] -> Select N_nod (2)/1
  Gain3/1 -> [p_r]
  [p0_r] -> Gain3/1
  [p_r] -> Density Look-up/1
  [h0_r] -> Mux1/1
  Select 1:(N-1)/1 -> Mux1/2
  [h_r] -> Select 1:(N-1)/1
  Refrigerant Enthalpy [J/kg]/1 -> Sum/2, [h_r]
  Gain9/1 -> Refrigerant Enthalpy [J/kg]/2
  Product2/1 -> Sum1/1
  [rho_r] -> Product2/2
  Constant1/1 -> Product2/3
  Sum1/1 -> Refrigerant Enthalpy [J/kg]/1
  Product1/1 -> Sum1/2
  Sum/1 -> Product1/2
  Product/1 -> Product1/1
  [W_r] -> Product/1
  [rho_r] -> Product/2
  Constant/1 -> Product/3
  Gain6/1 -> [rho_r]
  Gain1/1 -> Density Look-up/2
  Density Look-up/1 -> Gain6/1
  [p_r] -> Select N_nod (1)/1
  [W_r] -> Gain5/1
  Mux/1 -> "RF: (h2, p2, W2)"/1
  "RF: (h1, p1, W1)"/1 -> Demux/1
  Demux/2 -> [p0_r]
  [h_r] -> Gain1/1
  F0022_louverFinHTC.m/1 -> Product5/2, F0022_louverSurfaceEffectiveness.m/1
  Divide1/1 -> F0022_louverFinHTC.m/1
  Constant3/1 -> Divide1/2
  Constant11/1 -> Divide1/3
  Product5/1 -> [Q_wa]
  [T_w] -> Sum4/1
  Outer fin + tube surface/1 -> Product5/1
  [T_a] -> Sum4/2
  Sum4/1 -> Product5/4
  F0022_louverSurfaceEffectiveness.m/1 -> Product5/3
  Demux1/1 -> [T_a]
  Demux1/2 -> [p_a]
  [p_a] -> Mux3/2
  Demux1/3 -> Gain11/1
  [W_a] -> Divide1/1
  [W_r] -> Gain4/1
  Gain4/1 -> Heat Tranfer Coefficient - Refrigerant Side/1(W_r [kg/s])
  [p0_r] -> F0021_Tsat.m/1
  F0021_Tsat.m/1 -> Gain7/1
  Constant4/1 -> Gain9/1
  Constant9/1 -> Product4/3
  Gain12/1 -> Mux3/3
  Gain11/1 -> Saturation1/1
  [W_a] -> Gain12/1
  [T_a] -> Sum5/2
  Sum5/1 -> Mux3/1
  [Q_wa] -> Sum6/1
  Sum6/1 -> Divide2/1
  Constant2/1 -> Divide2/2
  [W_a] -> Divide2/3
  Divide2/1 -> Sum5/1
  Saturation1/1 -> [W_a]

== system component_lib/Thermal Systems/RF0013_calculateHeatflow ==
  "RF: (h1, p1, W1)" : Inport
  "RF: (h2, p2, W2)" : Inport  Port=2
  Demux : Demux  Outputs=3
  Demux1 : Demux  Outputs=3
  Product : Product
  Product1 : Product
  Sum : Sum  Inputs=|+-
  Terminator : Terminator
  Terminator1 : Terminator
  Q [J/s] : Outport
  wires:
  "RF: (h1, p1, W1)"/1 -> Demux/1
  "RF: (h2, p2, W2)"/1 -> Demux1/1
  Sum/1 -> Q [J/s]/1
  Demux/2 -> Terminator/1
  Demux1/2 -> Terminator1/1
  Demux/1 -> Product/1
  Demux/3 -> Product/2
  Demux1/1 -> Product1/1
  Demux1/3 -> Product1/2
  Product1/1 -> Sum/1
  Product/1 -> Sum/2

== system component_lib/Thermal Systems/RF0014_calculateVaporFraction ==
  "RF: (h, p, W)" : Inport
  Demux : Demux  Outputs=3
  Gain2 : Gain  Gain=par.M
  Vapor Fraction Look-up : Lookup_n-D  BreakpointsForDimension1=R1234yf_ph.p  BreakpointsForDimension2=R1234yf_ph.h  Table=R1234yf_ph.x  InternalRulePriority=Speed  RndMeth=Simplest
      settings: InputPortMap=u0,u1
  x [-] : Outport
  wires:
  Demux/2 -> [p]
  Gain2/1 -> Vapor Fraction Look-up/2
  [p] -> Vapor Fraction Look-up/1
  [h] -> Gain2/1
  Vapor Fraction Look-up/1 -> x [-]/1
  "RF: (h, p, W)"/1 -> Demux/1
  Demux/1 -> [h]
  Demux/3 -> [W]

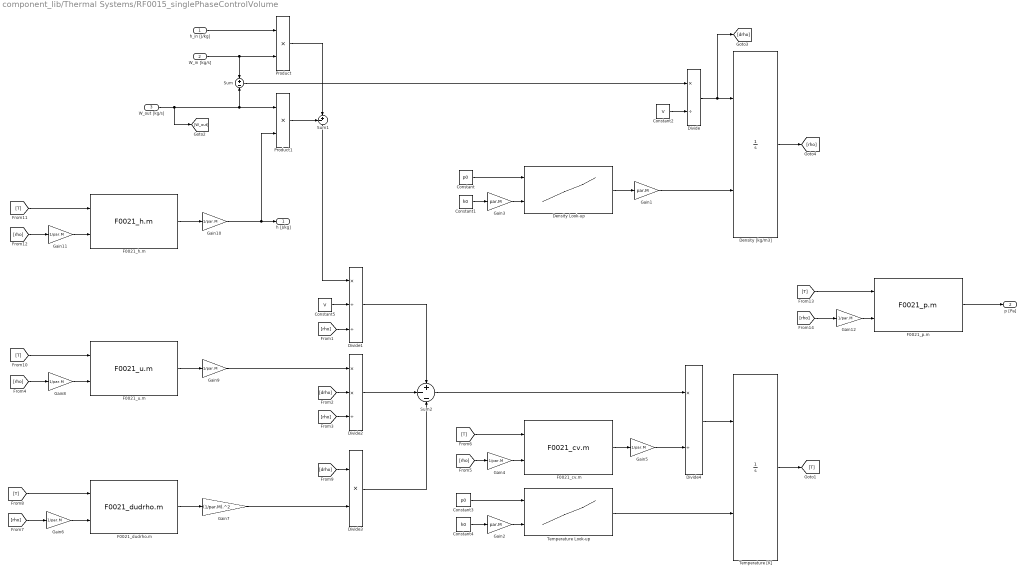
== system component_lib/Thermal Systems/RF0015_singlePhaseControlVolume ==
  h_in [J/kg] : Inport
  W_in [kg/s] : Inport  Port=2
  W_out [kg/s] : Inport  Port=3
  Constant : Constant  Value=p0
  Constant1 : Constant  Value=h0
  Constant2 : Constant  Value=V
  Constant3 : Constant  Value=p0
  Constant4 : Constant  Value=h0
  Constant5 : Constant  Value=V
  Density Look-up : Lookup_n-D  BreakpointsForDimension1=R1234yf_ph.p  BreakpointsForDimension2=R1234yf_ph.h  Table=R1234yf_ph.D  InternalRulePriority=Speed  RndMeth=Simplest
      settings: InputPortMap=u0,u1
  Density [kg/m3] : Integrator  InitialConditionSource=external  LimitOutput=on  LowerSaturationLimit=0
  Divide : Product  Inputs=*/
  Divide1 : Product  Inputs=*//
  Divide2 : Product  Inputs=**/
  Divide3 : Product  Inputs=**
  Divide4 : Product  Inputs=*/
  F0021_cv.m : base_lib/F0021_R1234yf/F0021_cv.m  SystemSampleTime=-1  VariantActivationTime=update diagram  Latency=0  AutoFrameSizeCalculation=off
      settings: LibrarySourceBlock=|
      | simulink/User-Defined
      | Functions/MATLAB Function
  F0021_dudrho.m : base_lib/F0021_R1234yf/F0021_dudrho.m  SystemSampleTime=-1  VariantActivationTime=update diagram  Latency=0  AutoFrameSizeCalculation=off
      settings: LibrarySourceBlock=|
      | simulink/User-Defined
      | Functions/MATLAB Function
  F0021_h.m : base_lib/F0021_R1234yf/F0021_h.m  SystemSampleTime=-1  VariantActivationTime=update diagram  Latency=0  AutoFrameSizeCalculation=off
      settings: LibrarySourceBlock=|
      | simulink/User-Defined
      | Functions/MATLAB Function
  F0021_p.m : base_lib/F0021_R1234yf/F0021_p.m  SystemSampleTime=-1  VariantActivationTime=update diagram  Latency=0  AutoFrameSizeCalculation=off
      settings: LibrarySourceBlock=|
      | simulink/User-Defined
      | Functions/MATLAB Function
  F0021_u.m : base_lib/F0021_R1234yf/F0021_u.m  SystemSampleTime=-1  VariantActivationTime=update diagram  Latency=0  AutoFrameSizeCalculation=off
      settings: LibrarySourceBlock=|
      | simulink/User-Defined
      | Functions/MATLAB Function
  Gain1 : Gain  Gain=par.M
  Gain{4..6,8..12} (8 alike) : Gain  Gain=1/par.M
  Gain2 : Gain  Gain=par.M
  Gain3 : Gain  Gain=par.M
  Gain7 : Gain  Gain=(1/par.M).^2
  Product : Product
  Product1 : Product
  Sum : Sum  Inputs=+|-
  Sum1 : Sum  Inputs=-+|
  Sum2 : Sum  Inputs=+--
  Temperature Look-up : Lookup_n-D  BreakpointsForDimension1=R1234yf_ph.p  BreakpointsForDimension2=R1234yf_ph.h  Table=R1234yf_ph.T  InternalRulePriority=Speed  RndMeth=Simplest
      settings: InputPortMap=u0,u1
  Temperature [K] : Integrator  InitialConditionSource=external  LimitOutput=on  LowerSaturationLimit=0
  h [J/kg] : Outport
  p [Pa] : Outport  Port=2
  wires:
  Density Look-up/1 -> Gain1/1
  Gain1/1 -> Density [kg/m3]/2
  Constant/1 -> Density Look-up/1
  Gain3/1 -> Density Look-up/2
  Constant1/1 -> Gain3/1
  Divide/1 -> Density [kg/m3]/1, [drho]
  Constant2/1 -> Divide/2
  Density [kg/m3]/1 -> [rho]
  Sum/1 -> Divide/1
  W_out [kg/s]/1 -> [W_out], Product1/1, Sum/2
  Temperature Look-up/1 -> Temperature [K]/2
  Gain2/1 -> Temperature Look-up/2
  Constant4/1 -> Gain2/1
  Constant3/1 -> Temperature Look-up/1
  Temperature [K]/1 -> [T]
  W_in [kg/s]/1 -> Product/2, Sum/1
  h_in [J/kg]/1 -> Product/1
  Gain10/1 -> h [J/kg]/1, Product1/2
  Product/1 -> Sum1/2
  Product1/1 -> Sum1/1
  Sum1/1 -> Divide1/1
  Constant5/1 -> Divide1/2
  [rho] -> Divide1/3
  [rho] -> Divide2/3
  [drho] -> Divide2/2
  Gain9/1 -> Divide2/1
  [rho] -> Gain4/1
  Gain4/1 -> F0021_cv.m/2
  F0021_cv.m/1 -> Gain5/1
  [T] -> F0021_cv.m/1
  Divide4/1 -> Temperature [K]/1
  Gain5/1 -> Divide4/2
  Sum2/1 -> Divide4/1
  Divide1/1 -> Sum2/1
  Divide2/1 -> Sum2/2
  Divide3/1 -> Sum2/3
  [rho] -> Gain6/1
  Gain6/1 -> F0021_dudrho.m/2
  [T] -> F0021_dudrho.m/1
  [drho] -> Divide3/1
  F0021_dudrho.m/1 -> Gain7/1
  Gain7/1 -> Divide3/2
  [T] -> F0021_u.m/1
  [rho] -> Gain8/1
  Gain8/1 -> F0021_u.m/2
  F0021_u.m/1 -> Gain9/1
  F0021_h.m/1 -> Gain10/1
  [rho] -> Gain11/1
  Gain11/1 -> F0021_h.m/2
  [T] -> F0021_h.m/1
  F0021_p.m/1 -> p [Pa]/1
  [rho] -> Gain12/1
  Gain12/1 -> F0021_p.m/2
  [T] -> F0021_p.m/1

== system component_lib/Thermal Systems/RF0016_split ==
  "A: (h, p, W)" : Inport
  split [-] : Inport  Port=2
  Constant : Constant
  Demux : Demux  Outputs=3
  Mux : Mux  Inputs=3
  Mux1 : Mux  Inputs=3
  Product : Product
  Product1 : Product
  Sum : Sum  Inputs=-+|
  "B: (h, p, Wb)" : Outport
  "C: (h, p, Wc)" : Outport  Port=2
  wires:
  "A: (h, p, W)"/1 -> Demux/1
  Mux/1 -> "B: (h, p, Wb)"/1
  Mux1/1 -> "C: (h, p, Wc)"/1
  Demux/3 -> [W]
  Demux/2 -> [p]
  Demux/1 -> [h]
  split [-]/1 -> Sum/1, Product/2
  [W] -> Product/1
  Constant/1 -> Sum/2
  Sum/1 -> Product1/2
  [W] -> Product1/1
  Product/1 -> Mux/3
  [p] -> Mux/2
  [p] -> Mux1/2
  [h] -> Mux/1
  [h] -> Mux1/1
  Product1/1 -> Mux1/3

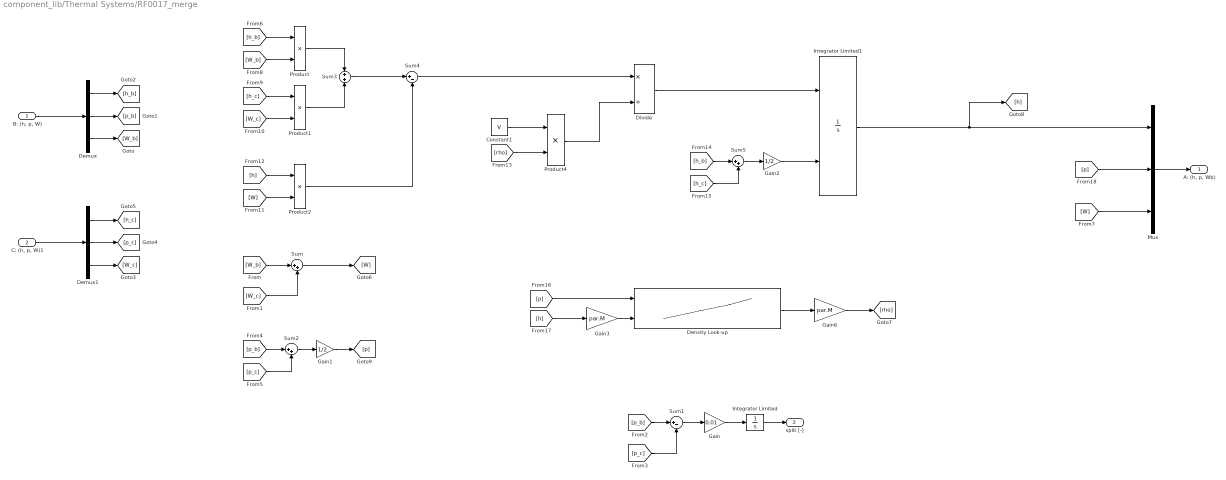
== system component_lib/Thermal Systems/RF0017_merge ==
  "B: (h, p, W)" : Inport
  "C: (h, p, W)1" : Inport  Port=2
  Constant1 : Constant  Value=V
  Demux : Demux  Outputs=3
  Demux1 : Demux  Outputs=3
  Density Look-up : Lookup_n-D  BreakpointsForDimension1=R1234yf_ph.p  BreakpointsForDimension2=R1234yf_ph.h  Table=R1234yf_ph.D  InternalRulePriority=Speed  RndMeth=Simplest
      settings: InputPortMap=u0,u1
  Divide : Product  Inputs=*/
  Gain : Gain  Gain=0.01
  Gain1 : Gain  Gain=1/2
  Gain2 : Gain  Gain=1/2
  Gain3 : Gain  Gain=par.M
  Gain6 : Gain  Gain=par.M
  Integrator Limited : Integrator  InitialCondition=0.5  LimitOutput=on  UpperSaturationLimit=1  LowerSaturationLimit=0
  Integrator Limited1 : Integrator  InitialConditionSource=external  InitialCondition=0.5  LimitOutput=on  LowerSaturationLimit=0
  Mux : Mux  Inputs=3
  Product{,1..2,4} (4 alike) : Product
  Sum : Sum  Inputs=|++
  Sum1 : Sum  Inputs=|+-
  Sum2 : Sum  Inputs=|++
  Sum3 : Sum  Inputs=+|+
  Sum4 : Sum  Inputs=|+-
  Sum5 : Sum  Inputs=|++
  "A: (h, p, Wb)" : Outport
  split [-] : Outport  Port=2
  wires:
  "B: (h, p, W)"/1 -> Demux/1
  Mux/1 -> "A: (h, p, Wb)"/1
  Demux/3 -> [W_b]
  Demux/2 -> [p_b]
  Demux/1 -> [h_b]
  Sum2/1 -> Gain1/1
  Demux1/1 -> [h_c]
  Demux1/3 -> [W_c]
  Demux1/2 -> [p_c]
  "C: (h, p, W)1"/1 -> Demux1/1
  [W_b] -> Sum/1
  [W_c] -> Sum/2
  [p_c] -> Sum1/2
  [p_b] -> Sum1/1
  Gain/1 -> Integrator Limited/1
  Sum1/1 -> Gain/1
  Integrator Limited/1 -> split [-]/1
  [p_b] -> Sum2/1
  [p_c] -> Sum2/2
  [h_b] -> Product/1
  [W_b] -> Product/2
  [W_c] -> Product1/2
  [h_c] -> Product1/1
  Product/1 -> Sum3/1
  Product1/1 -> Sum3/2
  Sum3/1 -> Sum4/1
  Sum/1 -> [W]
  [h] -> Product2/1
  [W] -> Product2/2
  [W] -> Mux/3
  Product2/1 -> Sum4/2
  Constant1/1 -> Product4/1
  [rho] -> Product4/2
  [h_b] -> Sum5/1
  [h_c] -> Sum5/2
  Sum5/1 -> Gain2/1
  Gain2/1 -> Integrator Limited1/2
  Divide/1 -> Integrator Limited1/1
  Sum4/1 -> Divide/1
  Product4/1 -> Divide/2
  Integrator Limited1/1 -> [h], Mux/1
  Density Look-up/1 -> Gain6/1
  [h] -> Gain3/1
  Gain3/1 -> Density Look-up/2
  Gain6/1 -> [rho]
  [p] -> Density Look-up/1
  Gain1/1 -> [p]
  [p] -> Mux/2

== system component_lib/Thermal Systems/RF0018_calculateTemperature ==
  "RF: (h, p, W)" : Inport
  Demux : Demux  Outputs=3
  Gain2 : Gain  Gain=par.M
  Temperature Look-up : Lookup_n-D  BreakpointsForDimension1=R1234yf_ph.p  BreakpointsForDimension2=R1234yf_ph.h  Table=R1234yf_ph.T  InternalRulePriority=Speed  RndMeth=Simplest
      settings: InputPortMap=u0,u1
  T [K] : Outport
  wires:
  "RF: (h, p, W)"/1 -> Demux/1
  Demux/2 -> [p]
  Gain2/1 -> Temperature Look-up/2
  [p] -> Temperature Look-up/1
  [h] -> Gain2/1
  Temperature Look-up/1 -> T [K]/1
  Demux/1 -> [h]
  Demux/3 -> [W]

== system component_lib/Thermal Systems/RF0019_receiver ==
  "RF: (h1, ~, W)" : Inport
  Constant1 : Constant  Commented=on  Value=V
  Constant2 : Constant  Value=0
  Constant3 : Constant  Value=p0
  Constant4 : Constant  Commented=on  Value=h0
  Demux : Demux  Outputs=3
  Density Look-up : Lookup_n-D  BreakpointsForDimension1=R1234yf_ph.p  BreakpointsForDimension2=R1234yf_ph.h  Table=R1234yf_ph.D  InternalRulePriority=Speed  RndMeth=Simplest
      settings: InputPortMap=u0,u1
  Divide : Product  Commented=on  Inputs=*/
  F0021_dliqsat.m : base_lib/F0021_R1234yf/F0021_dliqsat.m  Commented=on  SystemSampleTime=-1  VariantActivationTime=update diagram  Latency=0  AutoFrameSizeCalculation=off
      settings: LibrarySourceBlock=|
      | simulink/User-Defined
      | Functions/MATLAB Function
  F0021_h.m : base_lib/F0021_R1234yf/F0021_h.m  Commented=on  SystemSampleTime=-1  VariantActivationTime=update diagram  Latency=0  AutoFrameSizeCalculation=off
      settings: LibrarySourceBlock=|
      | simulink/User-Defined
      | Functions/MATLAB Function
  F0021_psat.m1 : base_lib/F0021_R1234yf/F0021_psat.m  SystemSampleTime=-1  VariantActivationTime=update diagram  Latency=0  AutoFrameSizeCalculation=off
      settings: LibrarySourceBlock=|
      | simulink/User-Defined
      | Functions/MATLAB Function
  From1 : From  Commented=on  GotoTag=rho
  From16 : From  Commented=on  GotoTag=T
  From2 : From  Commented=on  GotoTag=W
  From25 : From  Commented=on  GotoTag=rho_f
  From37 : From  Commented=on  GotoTag=T
  From4 : From  Commented=on  GotoTag=h_1
  From5 : From  Commented=on  GotoTag=W
  From6 : From  Commented=on  GotoTag=h_f
  Gain1 : Gain  Commented=on  Gain=1/par.M
  Gain16 : Gain  Commented=on  Gain=par.M
  Gain2 : Gain  Commented=on  Gain=1/par.M
  Gain3 : Gain  Gain=par.M
  Gain4 : Gain  Gain=par.M
  Gain5 : Gain  Gain=par.M
  Gain6 : Gain  Gain=p_gain
  Goto18 : Goto  Commented=on  GotoTag=rho_f
  Goto32 : Goto  Commented=on  GotoTag=h
  Goto4 : Goto  Commented=on  GotoTag=h_f
  Integrator : Integrator  InitialConditionSource=external  InitialCondition=p0
  Mux1 : Mux  Inputs=3
  Product1 : Product  Commented=on
  Product2 : Product  Commented=on
  Product3 : Product  Commented=on
  Specific Enthalpy [J/kg] : Integrator  Commented=on  InitialConditionSource=external  LimitOutput=on  LowerSaturationLimit=0
  Sum : Sum  Inputs=|+-
  Sum2 : Sum  Inputs=|++
  Sum3 : Sum  Commented=on  Inputs=+|-
  Temperature Look-up : Lookup_n-D  BreakpointsForDimension1=R1234yf_ph.p  BreakpointsForDimension2=R1234yf_ph.h  Table=R1234yf_ph.T  InternalRulePriority=Speed  RndMeth=Simplest
      settings: InputPortMap=u0,u1
  Terminator : Terminator
  "RF: (h2, p2, W)1" : Outport
  wires:
  F0021_h.m/1 -> Gain1/1
  Gain2/1 -> F0021_h.m/2
  From25/1 -> Gain2/1
  From16/1 -> F0021_h.m/1
  From37/1 -> F0021_dliqsat.m/1
  F0021_dliqsat.m/1 -> Gain16/1
  Gain16/1 -> Goto18/1
  From4/1 -> Product2/2
  From2/1 -> Product2/1
  Product2/1 -> Sum3/1
  From6/1 -> Product3/2
  Product3/1 -> Sum3/2
  From5/1 -> Product3/1
  Specific Enthalpy [J/kg]/1 -> Goto32/1
  [h] -> Gain4/1
  Gain4/1 -> Temperature Look-up/2
  [p] -> Temperature Look-up/1
  [T] -> F0021_psat.m1/1
  Constant1/1 -> Product1/2
  From1/1 -> Product1/1
  Density Look-up/1 -> Gain5/1
  Gain3/1 -> Density Look-up/2
  [p] -> Density Look-up/1
  [h] -> Gain3/1
  Gain5/1 -> [rho]
  Divide/1 -> Specific Enthalpy [J/kg]/1
  Sum3/1 -> Divide/1
  Product1/1 -> Divide/2
  Constant4/1 -> Specific Enthalpy [J/kg]/2
  "RF: (h1, ~, W)"/1 -> Demux/1
  Demux/1 -> [h]
  Demux/3 -> [W]
  Demux/2 -> Terminator/1
  Sum/1 -> Gain6/1
  Gain6/1 -> Integrator/1
  Integrator/1 -> Sum/2, [p]
  Constant3/1 -> Integrator/2
  Gain1/1 -> Goto4/1
  F0021_psat.m1/1 -> Sum/1
  Temperature Look-up/1 -> Sum2/1
  Constant2/1 -> Sum2/2
  Sum2/1 -> [T]
  [h] -> Mux1/1
  Mux1/1 -> "RF: (h2, p2, W)1"/1
  [p] -> Mux1/2
  [W] -> Mux1/3
